simulink model "CtrlStrct_VNT_Level2"  (R2018a)
settings: Solver=VariableStepAuto  StartTime=0.0  StopTime=10.0  FixedStep=sampletime  RelTol=1e-3  EnableMultiTasking=on
PreLoadFcn:
  | Controller_Struct_GoFrom_Scope_1_BusInfo
undefined symbols (not defined in the file or in its folder): canChannel
libraries: canlib x4, canmsglib x4, simulink x1
(part 1 of 2)
settings Model: Creator=IAEC nishito  LastModifiedBy=nishito
settings DataIOCC: LimitDataPoints=on  SaveFormat=Array  SaveOutput=off  SaveTime=off
settings OptimizationCC: DefaultParameterBehavior=Inlined  ExpressionDepthLimit=2147483647  LifeSpan=inf
settings DebuggingCC: UnderspecifiedInitializationDetection=Classic  MergeDetectMultiDrivingBlocksExec=none  SolverPrmCheckMsg=warning  InheritedTsInSrcMsg=none  FcnCallInpInsideContextMsg=warning  StateNameClashWarn=warning  SFUnexpectedBacktrackingDiag=warning  SFNoUnconditionalDefaultTransitionDiag=warning  SFExecutionAtInitializationDiag=none
settings HardwareCC: ProdBitPerPointer=32  ProdBitPerSizeT=32  ProdBitPerPtrDiffT=32  ProdLargestAtomicFloat=None  ProdIntDivRoundTo=Undefined  ProdEndianess=Unspecified  ProdWordSize=32  ProdHWDeviceType=32-bit Generic
settings ModelReferenceCC: ModelReferenceNumInstancesAllowed=Single  PropagateSignalLabelsOutOfModel=off
settings CodeAppCC: StateflowObjectComments=on
settings GRTTargetCC: TargetLangStandard=C89/C90 (ANSI)  GeneratePreprocessorConditionals=Disable all  CombineOutputUpdateFcns=off  GRTInterface=on
settings ConfigComp: CovMetricSettings=dw  CovHtmlReporting=on  CovSaveCumulativeToWorkspaceVar=on  CovSaveSingleToWorkspaceVar=on  CovExternalEMLEnable=off

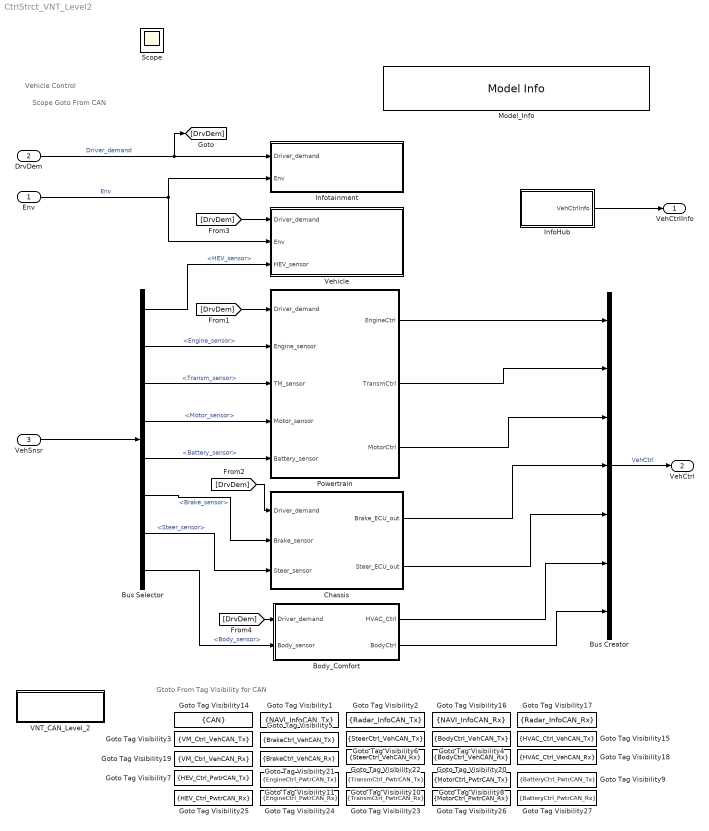
== system CtrlStrct_VNT_Level2 ==
  note: Scope Goto From CAN
  note: Gtoto From Tag Visibility for CAN
  note: Vehicle Control
  Env : Inport  OutDataTypeStr=Bus: Environment_Bus
      settings: AttributesFormatString=<%<OutDataTypeStr>>
  DrvDem : Inport  Port=2  OutDataTypeStr=Bus: Driver_demand_Bus
      settings: AttributesFormatString=%<OutDataTypeStr>
  VehSnsr : Inport  Port=3  OutDataTypeStr=Bus: Vehicle_sensor_Bus
      settings: AttributesFormatString=<%<OutDataTypeStr>>
  Body_Comfort : Subsystem
  Bus Creator : BusCreator  Inputs=7  OutDataTypeStr=Bus: Ctrl_intg_Bus
      settings: AttributesFormatString=%<OutDataTypeStr>
  Bus Selector : BusSelector  OutputSignals=HEV_sensor,Engine_sensor,Transm_sensor,Motor_sensor,Battery_sensor,Brake_sensor,Steer_sensor,Body_sensor
  Chassis : Subsystem
  Goto Tag Visibility1 : GotoTagVisibility  GotoTag=NAVI_InfoCAN_Tx
  Goto Tag Visibility10 : GotoTagVisibility  GotoTag=TransmCtrl_PwtrCAN_Tx
  Goto Tag Visibility11 : GotoTagVisibility  GotoTag=EngineCtrl_PwtrCAN_Tx
  Goto Tag Visibility14 : GotoTagVisibility  GotoTag=CAN
  Goto Tag Visibility15 : GotoTagVisibility  GotoTag=HVAC_Ctrl_VehCAN_Tx
  Goto Tag Visibility16 : GotoTagVisibility  GotoTag=NAVI_InfoCAN_Rx
  Goto Tag Visibility17 : GotoTagVisibility  GotoTag=Radar_InfoCAN_Rx
  Goto Tag Visibility18 : GotoTagVisibility  GotoTag=HVAC_Ctrl_VehCAN_Rx
  Goto Tag Visibility19 : GotoTagVisibility  GotoTag=VM_Ctrl_VehCAN_Rx
  Goto Tag Visibility2 : GotoTagVisibility  GotoTag=Radar_InfoCAN_Tx
  Goto Tag Visibility20 : GotoTagVisibility  GotoTag=BodyCtrl_VehCAN_Rx
  Goto Tag Visibility21 : GotoTagVisibility  GotoTag=BrakeCtrl_VehCAN_Rx
  Goto Tag Visibility22 : GotoTagVisibility  GotoTag=SteerCtrl_VehCAN_Rx
  Goto Tag Visibility23 : GotoTagVisibility  GotoTag=TransmCtrl_PwtrCAN_Rx
  Goto Tag Visibility24 : GotoTagVisibility  GotoTag=EngineCtrl_PwtrCAN_Rx
  Goto Tag Visibility25 : GotoTagVisibility  GotoTag=HEV_Ctrl_PwtrCAN_Rx
  Goto Tag Visibility26 : GotoTagVisibility  GotoTag=MotorCtrl_PwtrCAN_Rx
  Goto Tag Visibility27 : GotoTagVisibility  GotoTag=BatteryCtrl_PwtrCAN_Rx
  Goto Tag Visibility3 : GotoTagVisibility  GotoTag=VM_Ctrl_VehCAN_Tx
  Goto Tag Visibility4 : GotoTagVisibility  GotoTag=BodyCtrl_VehCAN_Tx
  Goto Tag Visibility5 : GotoTagVisibility  GotoTag=BrakeCtrl_VehCAN_Tx
  Goto Tag Visibility6 : GotoTagVisibility  GotoTag=SteerCtrl_VehCAN_Tx
  Goto Tag Visibility7 : GotoTagVisibility  GotoTag=HEV_Ctrl_PwtrCAN_Tx
  Goto Tag Visibility8 : GotoTagVisibility  GotoTag=MotorCtrl_PwtrCAN_Tx
  Goto Tag Visibility9 : GotoTagVisibility  GotoTag=BatteryCtrl_PwtrCAN_Tx
  InfoHub : Subsystem
  Infotainment : Subsystem
  Model_Info : simulink/Model-Wide Utilities/Model Info  Frame=on  DisplayStringWithTags=|  HorizontalTextAlignment=Left  LeftAlignmentValue=0.02
      | Version  %<ModelVersion>
      | LastModifided by %<LastModifiedBy>  Date %<LastModificationDate>
      | Description  %<Description>
  Powertrain : Subsystem
  VNT_CAN_Level_2 : Subsystem  VariantControl=VarObj_CanType_VNT_simu
  Vehicle : Subsystem
  VehCtrlInfo : Outport  OutDataTypeStr=Bus: IntgCtrl_Info_Bus
      settings: AttributesFormatString=<%<OutDataTypeStr>>
  VehCtrl : Outport  Port=2  OutDataTypeStr=Bus: Ctrl_intg_Bus
      settings: AttributesFormatString=<%<OutDataTypeStr>>
  Scope : Scope
  wires:
  InfoHub/1(VehCtrlInfo) -> VehCtrlInfo/1
  Chassis/2(Steer_ECU_out) -> Bus Creator/5
  Env/1 -> Vehicle/2(Env), Infotainment/2(Env)  "Env"
  Bus Creator/1 -> VehCtrl/1  "VehCtrl"
  [DrvDem] -> Powertrain/1(Driver_demand)
  Powertrain/3(MotorCtrl) -> Bus Creator/3
  Bus Selector/3 -> Powertrain/3(TM_sensor)  "<Transm_sensor>"
  Bus Selector/6 -> Chassis/2(Brake_sensor)  "<Brake_sensor>"
  Body_Comfort/2(BodyCtrl) -> Bus Creator/7
  Bus Selector/2 -> Powertrain/2(Engine_sensor)  "<Engine_sensor>"
  Powertrain/2(TransmCtrl) -> Bus Creator/2
  Chassis/1(Brake_ECU_out) -> Bus Creator/4
  VehSnsr/1 -> Bus Selector/1
  [DrvDem] -> Chassis/1(Driver_demand)
  Body_Comfort/1(HVAC_Ctrl) -> Bus Creator/6
  Bus Selector/1 -> Vehicle/3(HEV_sensor)  "<HEV_sensor>"
  Bus Selector/7 -> Chassis/3(Steer_sensor)  "<Steer_sensor>"
  Powertrain/1(EngineCtrl) -> Bus Creator/1
  [DrvDem] -> Vehicle/1(Driver_demand)
  Bus Selector/5 -> Powertrain/5(Battery_sensor)  "<Battery_sensor>"
  DrvDem/1 -> [DrvDem], Infotainment/1(Driver_demand)  "Driver_demand"
  Bus Selector/8 -> Body_Comfort/2(Body_sensor)  "<Body_sensor>"
  Bus Selector/4 -> Powertrain/4(Motor_sensor)  "<Motor_sensor>"
  [DrvDem] -> Body_Comfort/1(Driver_demand)

== system CtrlStrct_VNT_Level2/Body_Comfort ==
  note: Body Control
  Driver_demand : Inport
  Body_sensor : Inport  Port=2
  Body_Control : Subsystem
  HVAC_Control : Subsystem
  HVAC_Ctrl : Outport
  BodyCtrl : Outport  Port=2
  wires:
  Body_Control/1(BodyCtrl) -> BodyCtrl/1
  Driver_demand/1 -> HVAC_Control/1(Driver_demand), Body_Control/1(Driver_demand)
  Body_sensor/1 -> HVAC_Control/2(Body_sensor), Body_Control/2(Body_sensor)
  HVAC_Control/1(HVAC_Ctrl) -> HVAC_Ctrl/1

== system CtrlStrct_VNT_Level2/Chassis ==
  note: Chassis Control
  Driver_demand : Inport
  Brake_sensor : Inport  Port=2
  Steer_sensor : Inport  Port=3
  Brake_Control : Subsystem
  Steer_Control : Subsystem
  Brake_ECU_out : Outport
  Steer_ECU_out : Outport  Port=2
  wires:
  Driver_demand/1 -> Brake_Control/1(Driver_demand), Steer_Control/1(Driver_demand)
  Brake_Control/1(BrakeCtrl) -> Brake_ECU_out/1
  Brake_sensor/1 -> Brake_Control/2(Brake_sensor)
  Steer_Control/1(SteerCtrl) -> Steer_ECU_out/1
  Steer_sensor/1 -> Steer_Control/2(Steer_sensor)

== system CtrlStrct_VNT_Level2/InfoHub ==
  Bus Creator1 : BusCreator  Inputs=2
  Bus Selector : BusSelector  OutputSignals=VehCAN.BrakeCtrl_VehCAN_Tx.BrkCtrl_Vehicle_speed,PwtrCAN.EngineCtrl_PwtrCAN_Tx.EngCtrl_Engine_speed
  Terminator : Terminator
  Terminator1 : Terminator
  VehCtrlInfo : Outport
  wires:
  [HEV_ECU_Info] -> Bus Creator1/1
  [Engine_ECU_Info] -> Bus Creator1/2
  Bus Creator1/1 -> VehCtrlInfo/1  "VehCtrlInfo"
  [CAN] -> Bus Selector/1
  Bus Selector/2 -> Terminator/1  "<EngCtrl_Engine_speed>"
  Bus Selector/1 -> Terminator1/1  "<BrkCtrl_Vehicle_speed>"

== system CtrlStrct_VNT_Level2/Infotainment ==
  note: Infotainment
  Driver_demand : Inport
  Env : Inport  Port=2
  Navigation : Subsystem
  Radar_Detection : Subsystem
  wires:
  Env/1 -> Navigation/2(Env), Radar_Detection/2(Env)
  Driver_demand/1 -> Radar_Detection/1(Driver_demand), Navigation/1(Driver_demand)

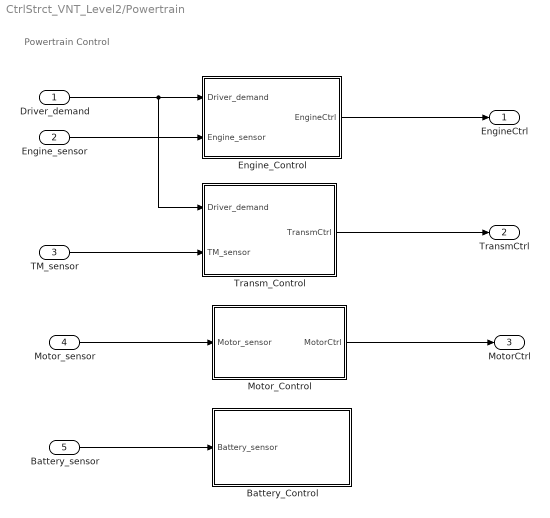
== system CtrlStrct_VNT_Level2/Powertrain ==
  note: Powertrain Control
  Driver_demand : Inport
  Engine_sensor : Inport  Port=2
  TM_sensor : Inport  Port=3
  Motor_sensor : Inport  Port=4
  Battery_sensor : Inport  Port=5
  Battery_Control : Subsystem
  Engine_Control : Subsystem
  Motor_Control : Subsystem
  Transm_Control : Subsystem
  EngineCtrl : Outport
  TransmCtrl : Outport  Port=2
  MotorCtrl : Outport  Port=3
  wires:
  Driver_demand/1 -> Transm_Control/1(Driver_demand), Engine_Control/1(Driver_demand)
  Motor_Control/1(MotorCtrl) -> MotorCtrl/1
  Motor_sensor/1 -> Motor_Control/1(Motor_sensor)
  Battery_sensor/1 -> Battery_Control/1(Battery_sensor)
  Engine_Control/1(EngineCtrl) -> EngineCtrl/1
  Engine_sensor/1 -> Engine_Control/2(Engine_sensor)
  Transm_Control/1(TransmCtrl) -> TransmCtrl/1
  TM_sensor/1 -> Transm_Control/2(TM_sensor)

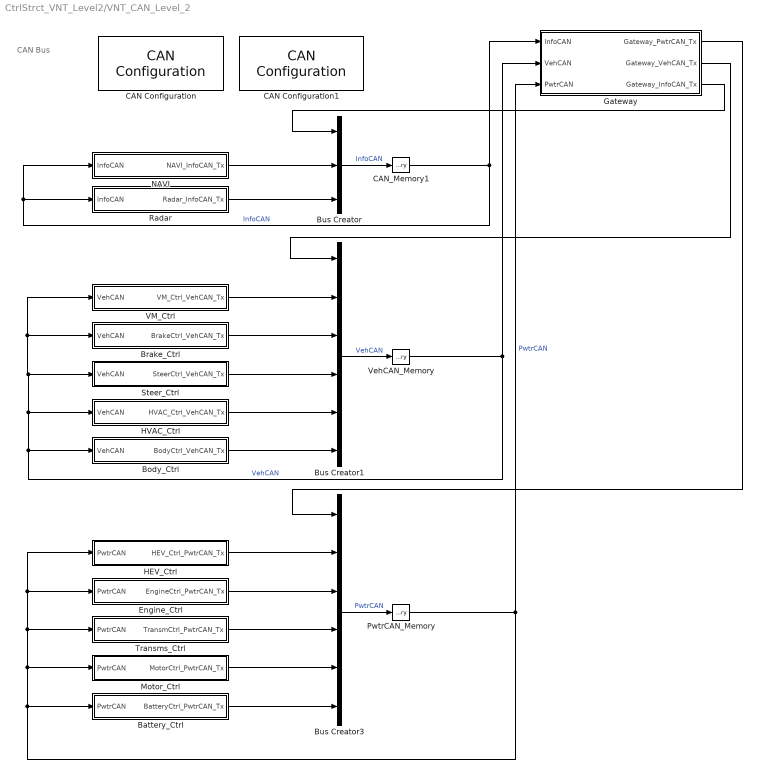
== system CtrlStrct_VNT_Level2/VNT_CAN_Level_2 ==
  note: CAN Bus
  Battery_Ctrl : Subsystem
  Body_Ctrl : Subsystem
  Brake_Ctrl : Subsystem
  Bus Creator : BusCreator  Inputs=3
  Bus Creator1 : BusCreator  Inputs=6
  Bus Creator3 : BusCreator  Inputs=6
  CAN Configuration : canlib/CAN Configuration  BlockHandle=38729.0009  DeviceMenu=MathWorks Virtual 1 (Channel 1)  Device=MathWorks Virtual 1 (Channel 1)  ObjConstructor=canChannel('MathWorks','Virtual 1',1)  BusSpeed=500000  EnableBitParameters=off  AckMode=Normal
      settings: SourceProductName=Vehicle Network Toolbox  SourceProductBaseCode=VN
  CAN Configuration1 : canlib/CAN Configuration  BlockHandle=38730.0009  DeviceMenu=MathWorks Virtual 1 (Channel 2)  Device=MathWorks Virtual 1 (Channel 2)  ObjConstructor=canChannel('MathWorks','Virtual 1',2)  BusSpeed=500000  EnableBitParameters=off  AckMode=Normal
      settings: SourceProductName=Vehicle Network Toolbox  SourceProductBaseCode=VN
  CAN_Memory1 : Memory
  Engine_Ctrl : Subsystem
  Gateway : Subsystem
  HEV_Ctrl : Subsystem
  HVAC_Ctrl : Subsystem
  Motor_Ctrl : Subsystem
  NAVI : Subsystem
  PwtrCAN_Memory : Memory
  Radar : Subsystem
  Steer_Ctrl : Subsystem
  Transms_Ctrl : Subsystem
  VM_Ctrl : Subsystem
  VehCAN_Memory : Memory
  wires:
  Radar/1(Radar_InfoCAN_Tx) -> Bus Creator/3
  NAVI/1(NAVI_InfoCAN_Tx) -> Bus Creator/2
  VM_Ctrl/1(VM_Ctrl_VehCAN_Tx) -> Bus Creator1/2
  Brake_Ctrl/1(BrakeCtrl_VehCAN_Tx) -> Bus Creator1/3
  Steer_Ctrl/1(SteerCtrl_VehCAN_Tx) -> Bus Creator1/4
  HVAC_Ctrl/1(HVAC_Ctrl_VehCAN_Tx) -> Bus Creator1/5
  Body_Ctrl/1(BodyCtrl_VehCAN_Tx) -> Bus Creator1/6
  Battery_Ctrl/1(BatteryCtrl_PwtrCAN_Tx) -> Bus Creator3/6
  Transms_Ctrl/1(TransmCtrl_PwtrCAN_Tx) -> Bus Creator3/4
  Motor_Ctrl/1(MotorCtrl_PwtrCAN_Tx) -> Bus Creator3/5
  Gateway/3(Gateway_InfoCAN_Tx) -> Bus Creator/1
  CAN_Memory1/1 -> NAVI/1(InfoCAN), Radar/1(InfoCAN), Gateway/1(InfoCAN)  "InfoCAN"
  Gateway/2(Gateway_VehCAN_Tx) -> Bus Creator1/1
  Gateway/1(Gateway_PwtrCAN_Tx) -> Bus Creator3/1
  PwtrCAN_Memory/1 -> Motor_Ctrl/1(PwtrCAN), Transms_Ctrl/1(PwtrCAN), Engine_Ctrl/1(PwtrCAN), HEV_Ctrl/1(PwtrCAN), Battery_Ctrl/1(PwtrCAN), Gateway/3(PwtrCAN)  "PwtrCAN"
  VehCAN_Memory/1 -> Body_Ctrl/1(VehCAN), HVAC_Ctrl/1(VehCAN), Brake_Ctrl/1(VehCAN), VM_Ctrl/1(VehCAN), Steer_Ctrl/1(VehCAN), Gateway/2(VehCAN)  "VehCAN"
  HEV_Ctrl/1(HEV_Ctrl_PwtrCAN_Tx) -> Bus Creator3/2
  Engine_Ctrl/1(EngineCtrl_PwtrCAN_Tx) -> Bus Creator3/3
  Bus Creator3/1 -> PwtrCAN_Memory/1  "PwtrCAN"
  Bus Creator/1 -> CAN_Memory1/1  "InfoCAN"
  Bus Creator1/1 -> VehCAN_Memory/1  "VehCAN"

== system CtrlStrct_VNT_Level2/Vehicle ==
  note: Vehicle Integrated Control
  Driver_demand : Inport
  Env : Inport  Port=2
  HEV_sensor : Inport  Port=3
  HEV_Control : Subsystem
  Vehicle_Motion_Control : Subsystem
  wires:
  Env/1 -> Vehicle_Motion_Control/1(Env)
  Driver_demand/1 -> HEV_Control/1(Driver_demand)
  HEV_sensor/1 -> HEV_Control/2(HEV_sensor)

== system CtrlStrct_VNT_Level2/Body_Comfort/Body_Control ==
  note: Body Control
  Driver_demand : Inport
  Body_sensor : Inport  Port=2
  BodyControlModule : ModelReference  ModelNameDialog=BodyCtrl_V1_1.slx  SimulationMode=Normal  ModelReferenceVersion=0.1.16
  Rate Transition1 : RateTransition  Deterministic=off
      settings: AttributesFormatString=<Deterministic=%<Deterministic>>
  Rate Transition2 : RateTransition  Deterministic=off
      settings: AttributesFormatString=<Deterministic=%<Deterministic>>
  Rate Transition4 : RateTransition  Deterministic=off
      settings: AttributesFormatString=<Deterministic=%<Deterministic>>
  BodyCtrl : Outport
  tag scope: BodyCtrl_VehCAN_Tx=scoped
  wires:
  Driver_demand/1 -> Rate Transition2/1
  Rate Transition2/1 -> BodyControlModule/1
  BodyControlModule/1 -> Rate Transition4/1
  [BodyCtrl_VehCAN_Rx] -> BodyControlModule/3
  BodyControlModule/2 -> [BodyCtrl_VehCAN_Tx]  "BodyCtrl_VehCAN_Tx"
  Rate Transition4/1 -> BodyCtrl/1  "BodyCtrl"
  Body_sensor/1 -> Rate Transition1/1
  Rate Transition1/1 -> BodyControlModule/2

== system CtrlStrct_VNT_Level2/Body_Comfort/HVAC_Control ==
  note: HVAC Control
  Driver_demand : Inport
  Body_sensor : Inport  Port=2
  Aircon_Control : ModelReference  ModelNameDialog=HVAC_Ctrl_V1_1.slx  SimulationMode=Normal  ModelReferenceVersion=0.1.22
  Rate Transition1 : RateTransition  Deterministic=off
      settings: AttributesFormatString=<Deterministic=%<Deterministic>>
  Rate Transition2 : RateTransition  Deterministic=off
      settings: AttributesFormatString=<Deterministic=%<Deterministic>>
  Rate Transition4 : RateTransition  Deterministic=off
      settings: AttributesFormatString=<Deterministic=%<Deterministic>>
  HVAC_Ctrl : Outport
  tag scope: HVAC_Ctrl_VehCAN_Tx=scoped
  wires:
  Rate Transition1/1 -> Aircon_Control/2
  Body_sensor/1 -> Rate Transition1/1
  Rate Transition4/1 -> HVAC_Ctrl/1  "HVAC_Ctrl"
  Aircon_Control/2 -> [HVAC_Ctrl_VehCAN_Tx]  "HVAC_Ctrl_VehCAN_Tx"
  [HVAC_Ctrl_VehCAN_Rx] -> Aircon_Control/3
  Aircon_Control/1 -> Rate Transition4/1
  Rate Transition2/1 -> Aircon_Control/1
  Driver_demand/1 -> Rate Transition2/1

== system CtrlStrct_VNT_Level2/Chassis/Brake_Control ==
  note: Brake Control
  Driver_demand : Inport
  Brake_sensor : Inport  Port=2
  Brake_Control : ModelReference  ModelNameDialog=BrakeCtrl_V1_1.slx  SimulationMode=Normal  ModelReferenceVersion=1.0.23
  Rate Transition1 : RateTransition  Deterministic=off
      settings: AttributesFormatString=<Deterministic=%<Deterministic>>
  Rate Transition2 : RateTransition  Deterministic=off
      settings: AttributesFormatString=<Deterministic=%<Deterministic>>
  Rate Transition4 : RateTransition  Deterministic=off
      settings: AttributesFormatString=<Deterministic=%<Deterministic>>
  Terminator : Terminator
  BrakeCtrl : Outport
  tag scope: BrakeCtrl_VehCAN_Tx=scoped
  wires:
  Rate Transition2/1 -> Brake_Control/2
  Driver_demand/1 -> Rate Transition1/1
  Rate Transition1/1 -> Brake_Control/1
  Brake_sensor/1 -> Rate Transition2/1
  Brake_Control/3 -> Terminator/1
  [BrakeCtrl_VehCAN_Rx] -> Brake_Control/3
  Rate Transition4/1 -> BrakeCtrl/1  "BrakeCtrl"
  Brake_Control/1 -> Rate Transition4/1
  Brake_Control/2 -> [BrakeCtrl_VehCAN_Tx]  "BrakeCtrl_VehCAN_Tx"

== system CtrlStrct_VNT_Level2/Chassis/Steer_Control ==
  note: Steering Control
  Driver_demand : Inport
  Steer_sensor : Inport  Port=2
  Rate Transition3 : RateTransition  Deterministic=off
      settings: AttributesFormatString=<Deterministic=%<Deterministic>>
  Rate Transition4 : RateTransition  Deterministic=off
      settings: AttributesFormatString=<Deterministic=%<Deterministic>>
  Rate Transition5 : RateTransition  Deterministic=off
      settings: AttributesFormatString=<Deterministic=%<Deterministic>>
  Steer_Control : ModelReference  ModelNameDialog=SteerCtrl_V1_1.slx  SimulationMode=Normal  ModelReferenceVersion=0.1.16
  SteerCtrl : Outport
  tag scope: SteerCtrl_VehCAN_Tx=scoped
  wires:
  Rate Transition4/1 -> Steer_Control/2
  Driver_demand/1 -> Rate Transition3/1
  Steer_Control/1 -> Rate Transition5/1
  Steer_sensor/1 -> Rate Transition4/1
  [SteerCtrl_VehCAN_Rx] -> Steer_Control/3
  Rate Transition3/1 -> Steer_Control/1
  Rate Transition5/1 -> SteerCtrl/1  "SteerCtrl"
  Steer_Control/2 -> [SteerCtrl_VehCAN_Tx]  "SteerCtrl_VehCAN_Tx"

== system CtrlStrct_VNT_Level2/Infotainment/Navigation ==
  note: Navigation
  Driver_demand : Inport
  Env : Inport  Port=2
  NAVI : ModelReference  ModelNameDialog=NAVI_V1_1.slx  SimulationMode=Normal  ModelReferenceVersion=0.1.17
  Rate Transition1 : RateTransition  Deterministic=off
      settings: AttributesFormatString=<Deterministic=%<Deterministic>>
  Rate Transition4 : RateTransition  Deterministic=off
      settings: AttributesFormatString=<Deterministic=%<Deterministic>>
  tag scope: NAVI_InfoCAN_Tx=scoped
  wires:
  Rate Transition1/1 -> NAVI/1
  Driver_demand/1 -> Rate Transition1/1
  [NAVI_InfoCAN_Rx] -> NAVI/3
  NAVI/1 -> [NAVI_InfoCAN_Tx]  "NAVI_InfoCAN_Tx"
  Env/1 -> Rate Transition4/1
  Rate Transition4/1 -> NAVI/2

== system CtrlStrct_VNT_Level2/Infotainment/Radar_Detection ==
  note: Radar Detection
  Driver_demand : Inport
  Env : Inport  Port=2
  Radar_Detection : ModelReference  ModelNameDialog=Radar_V1_1.slx  SimulationMode=Normal  ModelReferenceVersion=0.1.17
  Rate Transition1 : RateTransition  Deterministic=off
      settings: AttributesFormatString=<Deterministic=%<Deterministic>>
  Rate Transition4 : RateTransition  Deterministic=off
      settings: AttributesFormatString=<Deterministic=%<Deterministic>>
  tag scope: Radar_InfoCAN_Tx=scoped
  wires:
  Rate Transition1/1 -> Radar_Detection/2
  Env/1 -> Rate Transition1/1
  [Radar_InfoCAN_Rx] -> Radar_Detection/3
  Radar_Detection/1 -> [Radar_InfoCAN_Tx]  "Radar_InfoCAN_Tx"
  Driver_demand/1 -> Rate Transition4/1
  Rate Transition4/1 -> Radar_Detection/1

== system CtrlStrct_VNT_Level2/Powertrain/Battery_Control ==
  note: Battery Control
  Battery_sensor : Inport
  Battery_Control : ModelReference  ModelNameDialog=BatteryCtrl_V1_1.slx  SimulationMode=Normal  ModelReferenceVersion=0.1.22
  Rate Transition1 : RateTransition  Deterministic=off
      settings: AttributesFormatString=<Deterministic=%<Deterministic>>
  tag scope: BatteryCtrl_PwtrCAN_Tx=scoped
  wires:
  Battery_sensor/1 -> Rate Transition1/1
  [BatteryCtrl_PwtrCAN_Rx] -> Battery_Control/2
  Rate Transition1/1 -> Battery_Control/1
  Battery_Control/1 -> [BatteryCtrl_PwtrCAN_Tx]  "BatteryCtrl_PwtrCAN_Tx"

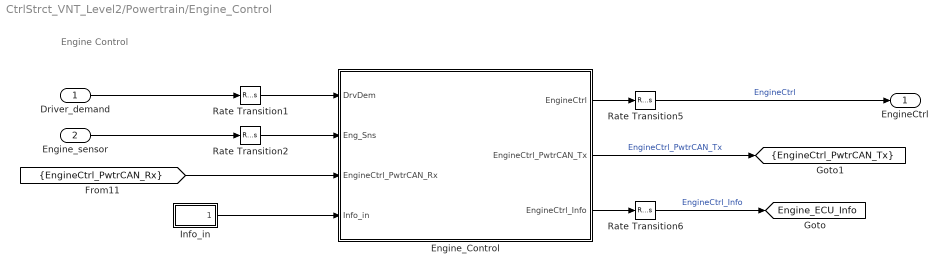
== system CtrlStrct_VNT_Level2/Powertrain/Engine_Control ==
  note: Engine Control
  Driver_demand : Inport
  Engine_sensor : Inport  Port=2
  Engine_Control : Subsystem  Variant=on
  Info_in : Subsystem
  Rate Transition{1..2,5..6} (4 alike) : RateTransition  Deterministic=off
      settings: AttributesFormatString=<Deterministic=%<Deterministic>>
  EngineCtrl : Outport
  tag scope: EngineCtrl_PwtrCAN_Tx=scoped, Engine_ECU_Info=global
  wires:
  Driver_demand/1 -> Rate Transition1/1
  Engine_sensor/1 -> Rate Transition2/1
  Rate Transition5/1 -> EngineCtrl/1  "EngineCtrl"
  Rate Transition6/1 -> [Engine_ECU_Info]  "EngineCtrl_Info"
  Engine_Control/2(" EngineCtrl_PwtrCAN_Tx") -> [EngineCtrl_PwtrCAN_Tx]  "EngineCtrl_PwtrCAN_Tx"
  Rate Transition1/1 -> Engine_Control/1("DrvDem ")
  Rate Transition2/1 -> Engine_Control/2("Eng_Sns ")
  [EngineCtrl_PwtrCAN_Rx] -> Engine_Control/3(EngineCtrl_PwtrCAN_Rx)
  Info_in/1(Info_in) -> Engine_Control/4("Info_in ")
  Engine_Control/1(" EngineCtrl") -> Rate Transition5/1
  Engine_Control/3(" EngineCtrl_Info") -> Rate Transition6/1

== system CtrlStrct_VNT_Level2/Powertrain/Motor_Control ==
  note: Motor Control
  Motor_sensor : Inport
  Motor_Control : ModelReference  ModelNameDialog=MotorCtrl_V1_1.slx  SimulationMode=Normal  ModelReferenceVersion=1.0.21
  Rate Transition1 : RateTransition  Deterministic=off
      settings: AttributesFormatString=<Deterministic=%<Deterministic>>
  Rate Transition3 : RateTransition  Deterministic=off
      settings: AttributesFormatString=<Deterministic=%<Deterministic>>
  Terminator : Terminator
  MotorCtrl : Outport
  tag scope: MotorCtrl_PwtrCAN_Tx=scoped
  wires:
  Rate Transition1/1 -> Motor_Control/1
  [MotorCtrl_PwtrCAN_Rx] -> Motor_Control/2
  Motor_sensor/1 -> Rate Transition1/1
  Motor_Control/3 -> Terminator/1
  Rate Transition3/1 -> MotorCtrl/1  "MotorCtrl"
  Motor_Control/1 -> Rate Transition3/1
  Motor_Control/2 -> [MotorCtrl_PwtrCAN_Tx]  "MotorCtrl_PwtrCAN_Tx"

== system CtrlStrct_VNT_Level2/Powertrain/Transm_Control ==
  note: Transmission Control
  Driver_demand : Inport
  TM_sensor : Inport  Port=2
  Rate Transition3 : RateTransition  Deterministic=off
      settings: AttributesFormatString=<Deterministic=%<Deterministic>>
  Rate Transition4 : RateTransition  Deterministic=off
      settings: AttributesFormatString=<Deterministic=%<Deterministic>>
  Rate Transition5 : RateTransition  Deterministic=off
      settings: AttributesFormatString=<Deterministic=%<Deterministic>>
  Terminator : Terminator
  Transm_ECU : ModelReference  ModelNameDialog=TransmCtrl_V1_1.slx  SimulationMode=Normal  ModelReferenceVersion=1.0.41
  TransmCtrl : Outport
  tag scope: TransmCtrl_PwtrCAN_Tx=scoped
  wires:
  Rate Transition4/1 -> Transm_ECU/2
  Transm_ECU/3 -> Terminator/1
  Driver_demand/1 -> Rate Transition3/1
  TM_sensor/1 -> Rate Transition4/1
  [TransmCtrl_PwtrCAN_Rx] -> Transm_ECU/3
  Rate Transition3/1 -> Transm_ECU/1
  Rate Transition5/1 -> TransmCtrl/1  "TransmCtrl"
  Transm_ECU/1 -> Rate Transition5/1
  Transm_ECU/2 -> [TransmCtrl_PwtrCAN_Tx]  "TransmCtrl_PwtrCAN_Tx"

== system CtrlStrct_VNT_Level2/VNT_CAN_Level_2/Battery_Ctrl ==
  note: Battery control
  note: CAN receive and transmit
  note: Battery Control
  PwtrCAN : Inport
  Bus Creator5 : BusCreator  Inputs=1
  Bus Selector : BusSelector  OutputSignals=HEV_Ctrl_PwtrCAN_Tx.HEVCtrl_Motor_torque_request
  Bus Selector1 : BusSelector  OutputSignals=BatCtrl_SOC
  Rate Transition1 : RateTransition  Deterministic=off
      settings: AttributesFormatString=<Deterministic=%<Deterministic>>
  Rate Transition2 : RateTransition  Deterministic=off
      settings: AttributesFormatString=<Deterministic=%<Deterministic>>
  Terminator : Terminator
  BatteryCtrl_PwtrCAN_Tx : Outport
  tag scope: BatteryCtrl_PwtrCAN_Rx=scoped
  wires:
  Bus Selector/1 -> Bus Creator5/1  "<HEVCtrl_Motor_torque_request>"
  PwtrCAN/1 -> Bus Selector/1
  Bus Creator5/1 -> Rate Transition1/1
  [BatteryCtrl_PwtrCAN_Tx] -> Rate Transition2/1, Bus Selector1/1
  Rate Transition1/1 -> [BatteryCtrl_PwtrCAN_Rx]  "BatteryCtrl_PwtrCAN_Rx"
  Rate Transition2/1 -> BatteryCtrl_PwtrCAN_Tx/1  "BatteryCtrl_PwtrCAN_Tx"
  Bus Selector1/1 -> Terminator/1  "<BatCtrl_SOC>"

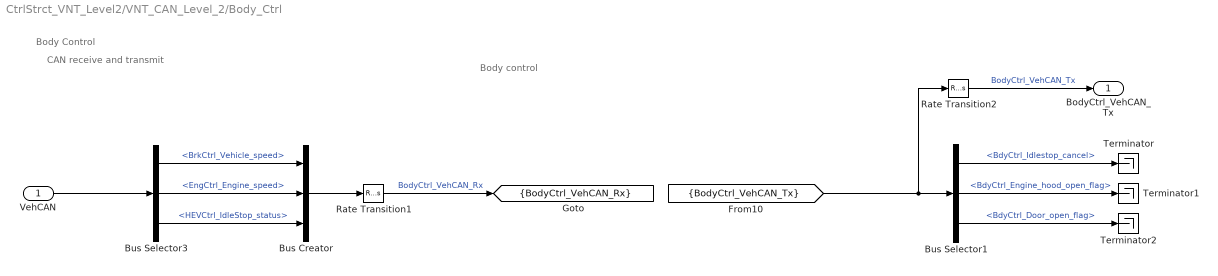
== system CtrlStrct_VNT_Level2/VNT_CAN_Level_2/Body_Ctrl ==
  note: Body Control
  note: CAN receive and transmit
  note: Body control
  VehCAN : Inport
  Bus Creator : BusCreator  Inputs=3
  Bus Selector1 : BusSelector  OutputSignals=BdyCtrl_Idlestop_cancel,BdyCtrl_Engine_hood_open_flag,BdyCtrl_Door_open_flag
  Bus Selector3 : BusSelector  OutputSignals=BrakeCtrl_VehCAN_Tx.BrkCtrl_Vehicle_speed,Gateway_VehCAN_Tx.EngCtrl_Engine_speed,Gateway_VehCAN_Tx.HEVCtrl_IdleStop_status
  Rate Transition1 : RateTransition  Deterministic=off
      settings: AttributesFormatString=<Deterministic=%<Deterministic>>
  Rate Transition2 : RateTransition  Deterministic=off
      settings: AttributesFormatString=<Deterministic=%<Deterministic>>
  Terminator : Terminator
  Terminator1 : Terminator
  Terminator2 : Terminator
  BodyCtrl_VehCAN_Tx : Outport
  tag scope: BodyCtrl_VehCAN_Rx=scoped
  wires:
  Bus Selector1/3 -> Terminator2/1  "<BdyCtrl_Door_open_flag>"
  Bus Selector1/1 -> Terminator/1  "<BdyCtrl_Idlestop_cancel>"
  Bus Selector1/2 -> Terminator1/1  "<BdyCtrl_Engine_hood_open_flag>"
  Rate Transition2/1 -> BodyCtrl_VehCAN_Tx/1  "BodyCtrl_VehCAN_Tx"
  Rate Transition1/1 -> [BodyCtrl_VehCAN_Rx]  "BodyCtrl_VehCAN_Rx"
  [BodyCtrl_VehCAN_Tx] -> Bus Selector1/1, Rate Transition2/1
  VehCAN/1 -> Bus Selector3/1
  Bus Creator/1 -> Rate Transition1/1
  Bus Selector3/2 -> Bus Creator/2  "<EngCtrl_Engine_speed>"
  Bus Selector3/1 -> Bus Creator/1  "<BrkCtrl_Vehicle_speed>"
  Bus Selector3/3 -> Bus Creator/3  "<HEVCtrl_IdleStop_status>"

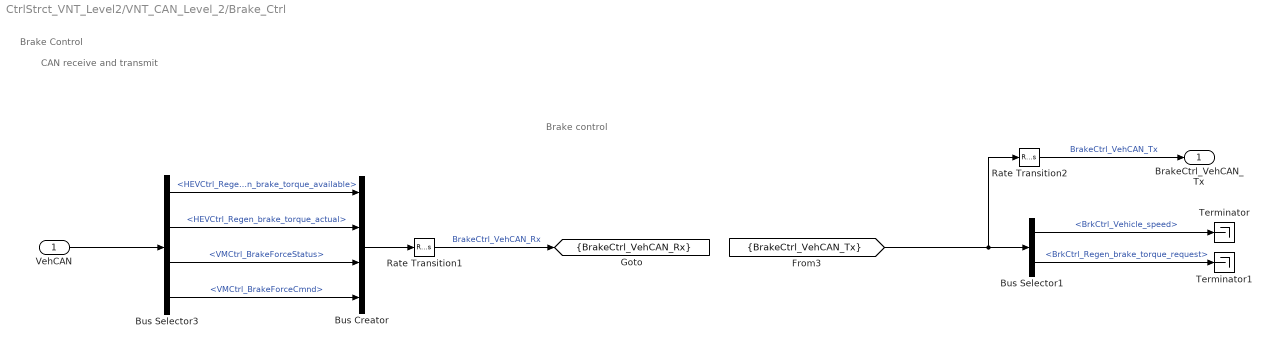
== system CtrlStrct_VNT_Level2/VNT_CAN_Level_2/Brake_Ctrl ==
  note: Brake Control
  note: CAN receive and transmit
  note: Brake control
  VehCAN : Inport
  Bus Creator : BusCreator  Inputs=4
  Bus Selector1 : BusSelector  OutputSignals=BrkCtrl_Vehicle_speed,BrkCtrl_Regen_brake_torque_request
  Bus Selector3 : BusSelector  OutputSignals=Gateway_VehCAN_Tx.HEVCtrl_Regen_brake_torque_available,Gateway_VehCAN_Tx.HEVCtrl_Regen_brake_torque_actual,VM_Ctrl_VehCAN_Tx.VMCtrl_BrakeForceStatus,VM_Ctrl_VehCAN_Tx.VMCtrl_BrakeForceCmnd
  Rate Transition1 : RateTransition  Deterministic=off
      settings: AttributesFormatString=<Deterministic=%<Deterministic>>
  Rate Transition2 : RateTransition  Deterministic=off
      settings: AttributesFormatString=<Deterministic=%<Deterministic>>
  Terminator : Terminator
  Terminator1 : Terminator
  BrakeCtrl_VehCAN_Tx : Outport
  tag scope: BrakeCtrl_VehCAN_Rx=scoped
  wires:
  Bus Selector1/1 -> Terminator/1  "<BrkCtrl_Vehicle_speed>"
  Bus Selector1/2 -> Terminator1/1  "<BrkCtrl_Regen_brake_torque_request>"
  Rate Transition2/1 -> BrakeCtrl_VehCAN_Tx/1  "BrakeCtrl_VehCAN_Tx"
  Rate Transition1/1 -> [BrakeCtrl_VehCAN_Rx]  "BrakeCtrl_VehCAN_Rx"
  [BrakeCtrl_VehCAN_Tx] -> Bus Selector1/1, Rate Transition2/1
  VehCAN/1 -> Bus Selector3/1
  Bus Creator/1 -> Rate Transition1/1
  Bus Selector3/3 -> Bus Creator/3  "<VMCtrl_BrakeForceStatus>"
  Bus Selector3/2 -> Bus Creator/2  "<HEVCtrl_Regen_brake_torque_actual>"
  Bus Selector3/4 -> Bus Creator/4  "<VMCtrl_BrakeForceCmnd>"
  Bus Selector3/1 -> Bus Creator/1  "<HEVCtrl_Regen_brake_torque_available>"

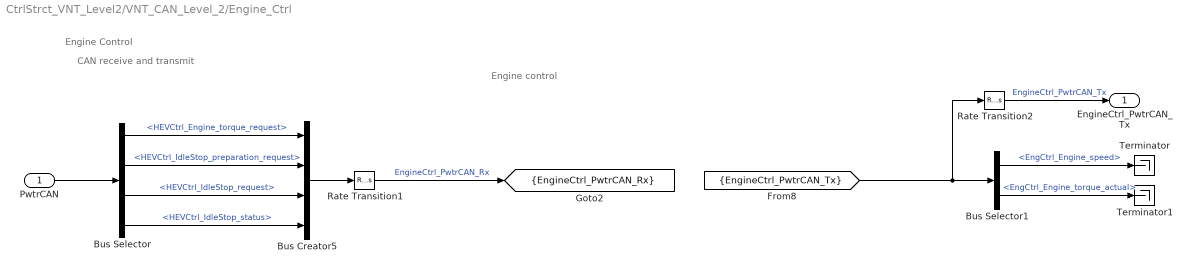
== system CtrlStrct_VNT_Level2/VNT_CAN_Level_2/Engine_Ctrl ==
  note: Engine control
  note: Engine Control
  note: CAN receive and transmit
  PwtrCAN : Inport
  Bus Creator5 : BusCreator  Inputs=4
  Bus Selector : BusSelector  OutputSignals=HEV_Ctrl_PwtrCAN_Tx.HEVCtrl_Engine_torque_request,HEV_Ctrl_PwtrCAN_Tx.HEVCtrl_IdleStop_preparation_request,HEV_Ctrl_PwtrCAN_Tx.HEVCtrl_IdleStop_request,HEV_Ctrl_PwtrCAN_Tx.HEVCtrl_IdleStop_status
  Bus Selector1 : BusSelector  OutputSignals=EngCtrl_Engine_speed,EngCtrl_Engine_torque_actual
  Rate Transition1 : RateTransition  Deterministic=off
      settings: AttributesFormatString=<Deterministic=%<Deterministic>>
  Rate Transition2 : RateTransition  Deterministic=off
      settings: AttributesFormatString=<Deterministic=%<Deterministic>>
  Terminator : Terminator
  Terminator1 : Terminator
  EngineCtrl_PwtrCAN_Tx : Outport
  tag scope: EngineCtrl_PwtrCAN_Rx=scoped
  wires:
  Bus Selector/1 -> Bus Creator5/1  "<HEVCtrl_Engine_torque_request>"
  Bus Selector/3 -> Bus Creator5/3  "<HEVCtrl_IdleStop_request>"
  Bus Selector/4 -> Bus Creator5/4  "<HEVCtrl_IdleStop_status>"
  Bus Selector/2 -> Bus Creator5/2  "<HEVCtrl_IdleStop_preparation_request>"
  [EngineCtrl_PwtrCAN_Tx] -> Rate Transition2/1, Bus Selector1/1
  PwtrCAN/1 -> Bus Selector/1
  Bus Creator5/1 -> Rate Transition1/1
  Rate Transition1/1 -> [EngineCtrl_PwtrCAN_Rx]  "EngineCtrl_PwtrCAN_Rx"
  Rate Transition2/1 -> EngineCtrl_PwtrCAN_Tx/1  "EngineCtrl_PwtrCAN_Tx"
  Bus Selector1/2 -> Terminator1/1  "<EngCtrl_Engine_torque_actual>"
  Bus Selector1/1 -> Terminator/1  "<EngCtrl_Engine_speed>"

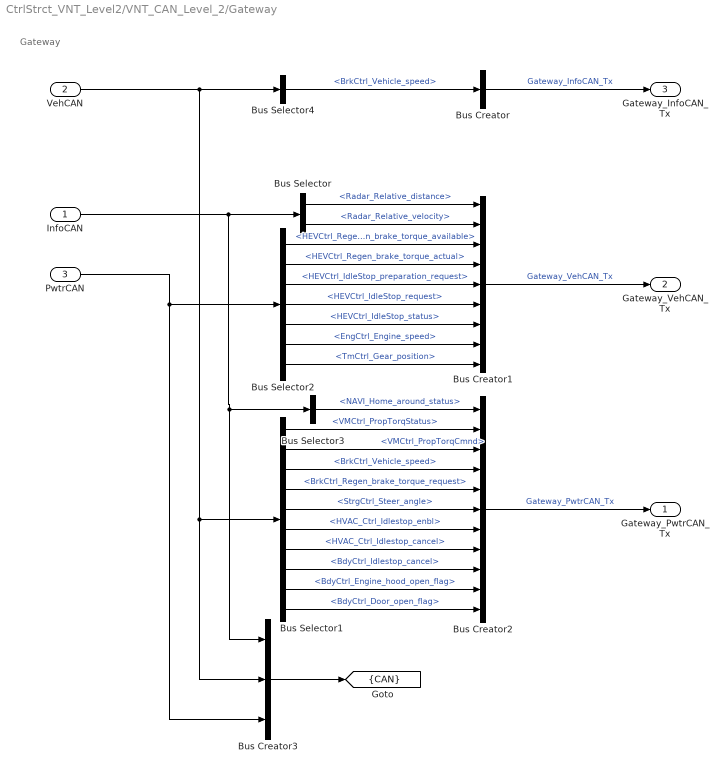
== system CtrlStrct_VNT_Level2/VNT_CAN_Level_2/Gateway ==
  note: Gateway
  InfoCAN : Inport
  VehCAN : Inport  Port=2
  PwtrCAN : Inport  Port=3
  Bus Creator : BusCreator  Inputs=1  OutDataTypeStr=Bus: Gateway_InfoCAN_Tx_Bus
      settings: AttributesFormatString=<%<OutDataTypeStr>>
  Bus Creator1 : BusCreator  Inputs=9  OutDataTypeStr=Bus: Gateway_VehCAN_Tx_Bus
      settings: AttributesFormatString=<%<OutDataTypeStr>>
  Bus Creator2 : BusCreator  Inputs=11  OutDataTypeStr=Bus: Gateway_PwtrCAN_Tx_Bus
      settings: AttributesFormatString=<%<OutDataTypeStr>>
  Bus Creator3 : BusCreator  Inputs=3
  Bus Selector : BusSelector  OutputSignals=Radar_InfoCAN_Tx.Radar_Relative_distance,Radar_InfoCAN_Tx.Radar_Relative_velocity
  Bus Selector1 : BusSelector  OutputSignals=VM_Ctrl_VehCAN_Tx.VMCtrl_PropTorqStatus,VM_Ctrl_VehCAN_Tx.VMCtrl_PropTorqCmnd,BrakeCtrl_VehCAN_Tx.BrkCtrl_Vehicle_speed,BrakeCtrl_VehCAN_Tx.BrkCtrl_Regen_brake_torque_request,SteerCtrl_VehCAN_Tx.StrgCtrl_Steer_angle,HVAC_Ctrl_VehCAN_Tx.HVAC_Ctrl_Idlestop_enbl,HVAC_Ctrl_VehCAN_Tx.HVAC_Ctrl_Idlestop_cancel,BodyCtrl_VehCAN_Tx.BdyCtrl_Idlestop_cancel,BodyCtrl_VehCAN_Tx.BdyCtrl_Engine_hood_open_flag,BodyCtrl_VehCAN_Tx.BdyCtrl_Door_open_flag
  Bus Selector2 : BusSelector  OutputSignals=HEV_Ctrl_PwtrCAN_Tx.HEVCtrl_Regen_brake_torque_available,HEV_Ctrl_PwtrCAN_Tx.HEVCtrl_Regen_brake_torque_actual,HEV_Ctrl_PwtrCAN_Tx.HEVCtrl_IdleStop_preparation_request,HEV_Ctrl_PwtrCAN_Tx.HEVCtrl_IdleStop_request,HEV_Ctrl_PwtrCAN_Tx.HEVCtrl_IdleStop_status,EngineCtrl_PwtrCAN_Tx.EngCtrl_Engine_speed,TransmCtrl_PwtrCAN_Tx.TmCtrl_Gear_position
  Bus Selector3 : BusSelector  OutputSignals=NAVI_InfoCAN_Tx.NAVI_Home_around_status
  Bus Selector4 : BusSelector  OutputSignals=BrakeCtrl_VehCAN_Tx.BrkCtrl_Vehicle_speed
  Gateway_PwtrCAN_Tx : Outport
  Gateway_VehCAN_Tx : Outport  Port=2
  Gateway_InfoCAN_Tx : Outport  Port=3
  tag scope: CAN=scoped
  wires:
  Bus Creator3/1 -> [CAN]
  Bus Creator/1 -> Gateway_InfoCAN_Tx/1  "Gateway_InfoCAN_Tx"
  Bus Selector4/1 -> Bus Creator/1  "<BrkCtrl_Vehicle_speed>"
  Bus Selector2/7 -> Bus Creator1/9  "<TmCtrl_Gear_position>"
  Bus Selector2/6 -> Bus Creator1/8  "<EngCtrl_Engine_speed>"
  Bus Selector2/2 -> Bus Creator1/4  "<HEVCtrl_Regen_brake_torque_actual>"
  Bus Selector2/1 -> Bus Creator1/3  "<HEVCtrl_Regen_brake_torque_available>"
  Bus Creator2/1 -> Gateway_PwtrCAN_Tx/1  "Gateway_PwtrCAN_Tx"
  Bus Selector1/10 -> Bus Creator2/11  "<BdyCtrl_Door_open_flag>"
  Bus Selector1/9 -> Bus Creator2/10  "<BdyCtrl_Engine_hood_open_flag>"
  Bus Selector1/8 -> Bus Creator2/9  "<BdyCtrl_Idlestop_cancel>"
  Bus Selector1/7 -> Bus Creator2/8  "<HVAC_Ctrl_Idlestop_cancel>"
  Bus Selector1/6 -> Bus Creator2/7  "<HVAC_Ctrl_Idlestop_enbl>"
  Bus Selector1/5 -> Bus Creator2/6  "<StrgCtrl_Steer_angle>"
  Bus Selector1/4 -> Bus Creator2/5  "<BrkCtrl_Regen_brake_torque_request>"
  Bus Selector1/3 -> Bus Creator2/4  "<BrkCtrl_Vehicle_speed>"
  Bus Selector3/1 -> Bus Creator2/1  "<NAVI_Home_around_status>"
  Bus Selector/2 -> Bus Creator1/2  "<Radar_Relative_velocity>"
  Bus Selector/1 -> Bus Creator1/1  "<Radar_Relative_distance>"
  InfoCAN/1 -> Bus Selector/1, Bus Selector3/1, Bus Creator3/1
  PwtrCAN/1 -> Bus Creator3/3, Bus Selector2/1
  Bus Creator1/1 -> Gateway_VehCAN_Tx/1  "Gateway_VehCAN_Tx"
  VehCAN/1 -> Bus Selector4/1, Bus Selector1/1, Bus Creator3/2
  Bus Selector1/1 -> Bus Creator2/2  "<VMCtrl_PropTorqStatus>"
  Bus Selector1/2 -> Bus Creator2/3  "<VMCtrl_PropTorqCmnd>"
  Bus Selector2/3 -> Bus Creator1/5  "<HEVCtrl_IdleStop_preparation_request>"
  Bus Selector2/4 -> Bus Creator1/6  "<HEVCtrl_IdleStop_request>"
  Bus Selector2/5 -> Bus Creator1/7  "<HEVCtrl_IdleStop_status>"

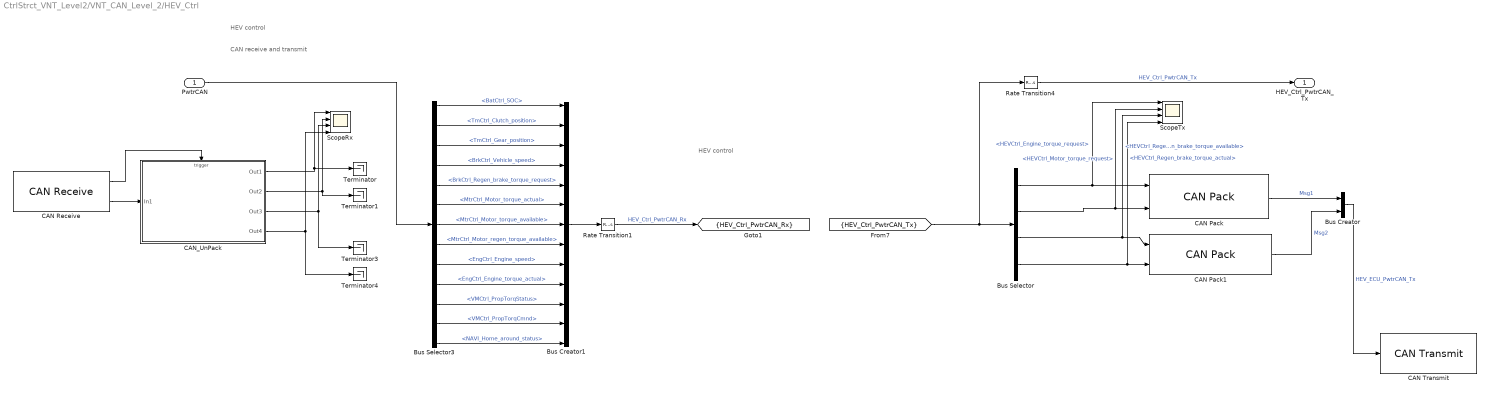
== system CtrlStrct_VNT_Level2/VNT_CAN_Level_2/HEV_Ctrl ==
  note: HEV control
  note: HEV control
  note: CAN receive and transmit
  PwtrCAN : Inport
  Bus Creator : BusCreator  Inputs=2
  Bus Creator1 : BusCreator  Inputs=13
  Bus Selector : BusSelector  OutputSignals=HEVCtrl_Engine_torque_request,HEVCtrl_Motor_torque_request,HEVCtrl_Regen_brake_torque_available,HEVCtrl_Regen_brake_torque_actual
  Bus Selector3 : BusSelector  OutputSignals=BatteryCtrl_PwtrCAN_Tx.BatCtrl_SOC,TransmCtrl_PwtrCAN_Tx.TmCtrl_Clutch_position,TransmCtrl_PwtrCAN_Tx.TmCtrl_Gear_position,Gateway_PwtrCAN_Tx.BrkCtrl_Vehicle_speed,Gateway_PwtrCAN_Tx.BrkCtrl_Regen_brake_torque_request,MotorCtrl_PwtrCAN_Tx.MtrCtrl_Motor_torque_actual,MotorCtrl_PwtrCAN_Tx.MtrCtrl_Motor_torque_available,MotorCtrl_PwtrCAN_Tx.MtrCtrl_Motor_regen_torque_available,EngineCtrl_PwtrCAN_Tx.EngCtrl_Engine_speed,EngineCtrl_PwtrCAN_Tx.EngCtrl_Engine_torque_actual,Gateway_PwtrCAN_Tx.VMCtrl_PropTorqStatus,Gateway_PwtrCAN_Tx.VMCtrl_PropTorqCmnd,Gateway_PwtrCAN_Tx.NAVI_Home_around_status
  CAN Pack : canmsglib/CAN Pack  MsgList=(none)  MsgName=CAN Msg1  MsgIDType=Standard (11-bit identifier)  MsgIdentifier=10  MsgLength=8  SignalInfo=Signal1$0$32$1$3$1$0$1$0$-Inf$Inf$#Signal2$32$32$1$3$1$0$1$0$-Inf$Inf$#  NSignals=2  StartBits=str2num('[int32(0);int32(32)]')  SignalSizes=str2num('[int32(32);int32(32)]')  ByteOrders=str2num('[int32(1);int32(1)]')  DataTypes=str2num('[int32(3);int32(3)]')  MultiplexTypes=str2num('[int32(1);int32(1)]')  MultiplexValues=str2num('[double(0);double(0)]')  Factors=str2num('[double(1);double(1)]')  Offsets=str2num('[double(0);double(0)]')  Minimums=str2num('[double(-Inf);double(-Inf)]')  Maximums=str2num('[double(Inf);double(Inf)]')  Remote=off  ApplyMinMax=off  BusOutput=off
      settings: SourceProductName=Simulink Real-Time  SourceProductBaseCode=XP  DataFormat=manually specified signals
  CAN Pack1 : canmsglib/CAN Pack  MsgList=(none)  MsgName=CAN Msg2  MsgIDType=Standard (11-bit identifier)  MsgIdentifier=20  MsgLength=8  SignalInfo=Signal1$0$32$1$3$1$0$1$0$-Inf$Inf$#Signal2$32$32$1$3$1$0$1$0$-Inf$Inf$#  NSignals=2  StartBits=str2num('[int32(0);int32(32)]')  SignalSizes=str2num('[int32(32);int32(32)]')  ByteOrders=str2num('[int32(1);int32(1)]')  DataTypes=str2num('[int32(3);int32(3)]')  MultiplexTypes=str2num('[int32(1);int32(1)]')  MultiplexValues=str2num('[double(0);double(0)]')  Factors=str2num('[double(1);double(1)]')  Offsets=str2num('[double(0);double(0)]')  Minimums=str2num('[double(-Inf);double(-Inf)]')  Maximums=str2num('[double(Inf);double(Inf)]')  Remote=off  ApplyMinMax=off  BusOutput=off
      settings: SourceProductName=Simulink Real-Time  SourceProductBaseCode=XP  DataFormat=manually specified signals
  CAN Receive : canlib/CAN Receive  BlockHandle=38824.0009  DeviceMenu=MathWorks Virtual 1 (Channel 1)  Device=MathWorks Virtual 1 (Channel 1)  ObjConstructor=canChannel('MathWorks','Virtual 1',1)  EnableStandardIDsFilter=off  StandardIDs=0  EnableExtendedIDsFilter=off  ExtendedIDs=0  SampleTime=0.01  MsgsPerTimestep=all  StdIDsCombo=Allow all  ExtIDsCombo=Allow all  InternalFilterUpdateStatus=off  BusOutput=off
      settings: SourceProductName=Vehicle Network Toolbox  SourceProductBaseCode=VN
  CAN Transmit : canlib/CAN Transmit  BlockHandle=38825.0009  DeviceMenu=MathWorks Virtual 1 (Channel 1)  Device=MathWorks Virtual 1 (Channel 1)  ObjConstructor=canChannel('MathWorks','Virtual 1',1)  EnablePeriodicTransmit=on  MessagePeriod=0.01
      settings: SourceProductName=Vehicle Network Toolbox  SourceProductBaseCode=VN
  CAN_UnPack : Subsystem
  Rate Transition1 : RateTransition  Deterministic=off
      settings: AttributesFormatString=<Deterministic=%<Deterministic>>
  Rate Transition4 : RateTransition  Deterministic=off
      settings: AttributesFormatString=<Deterministic=%<Deterministic>>
  ScopeRx : Scope  NumInputPorts=4
  ScopeTx : Scope  NumInputPorts=4
  Terminator{,1,3..4} (4 alike) : Terminator
  HEV_Ctrl_PwtrCAN_Tx : Outport
  tag scope: HEV_Ctrl_PwtrCAN_Rx=scoped
  wires:
  Bus Selector3/1 -> Bus Creator1/1  "<BatCtrl_SOC>"
  Bus Selector3/9 -> Bus Creator1/9  "<EngCtrl_Engine_speed>"
  Bus Selector3/8 -> Bus Creator1/8  "<MtrCtrl_Motor_regen_torque_available>"
  Bus Selector3/3 -> Bus Creator1/3  "<TmCtrl_Gear_position>"
  PwtrCAN/1 -> Bus Selector3/1
  Bus Selector3/6 -> Bus Creator1/6  "<MtrCtrl_Motor_torque_actual>"
  Bus Selector3/10 -> Bus Creator1/10  "<EngCtrl_Engine_torque_actual>"
  Bus Selector3/4 -> Bus Creator1/4  "<BrkCtrl_Vehicle_speed>"
  Bus Selector3/2 -> Bus Creator1/2  "<TmCtrl_Clutch_position>"
  Bus Selector3/7 -> Bus Creator1/7  "<MtrCtrl_Motor_torque_available>"
  Bus Selector3/5 -> Bus Creator1/5  "<BrkCtrl_Regen_brake_torque_request>"
  Bus Selector3/12 -> Bus Creator1/12  "<VMCtrl_PropTorqCmnd>"
  Bus Selector3/13 -> Bus Creator1/13  "<NAVI_Home_around_status>"
  Bus Selector3/11 -> Bus Creator1/11  "<VMCtrl_PropTorqStatus>"
  CAN Receive/1 -> CAN_UnPack/Trigger
  CAN Receive/2 -> CAN_UnPack/1(In1)
  CAN_UnPack/1(Out1) -> ScopeRx/1, Terminator/1
  CAN_UnPack/2(Out2) -> ScopeRx/2, Terminator1/1
  CAN_UnPack/4(Out4) -> ScopeRx/4, Terminator4/1
  CAN_UnPack/3(Out3) -> ScopeRx/3, Terminator3/1
  Bus Creator1/1 -> Rate Transition1/1
  Bus Creator/1 -> CAN Transmit/1  "HEV_ECU_PwtrCAN_Tx"
  CAN Pack1/1 -> Bus Creator/2  "Msg2"
  CAN Pack/1 -> Bus Creator/1  "Msg1"
  Bus Selector/4 -> CAN Pack1/2, ScopeTx/4  "<HEVCtrl_Regen_brake_torque_actual>"
  Bus Selector/3 -> ScopeTx/3, CAN Pack1/1  "<HEVCtrl_Regen_brake_torque_available>"
  Bus Selector/2 -> ScopeTx/2, CAN Pack/2  "<HEVCtrl_Motor_torque_request>"
  Bus Selector/1 -> ScopeTx/1, CAN Pack/1  "<HEVCtrl_Engine_torque_request>"
  [HEV_Ctrl_PwtrCAN_Tx] -> Rate Transition4/1, Bus Selector/1
  Rate Transition4/1 -> HEV_Ctrl_PwtrCAN_Tx/1  "HEV_Ctrl_PwtrCAN_Tx"
  Rate Transition1/1 -> [HEV_Ctrl_PwtrCAN_Rx]  "HEV_Ctrl_PwtrCAN_Rx"

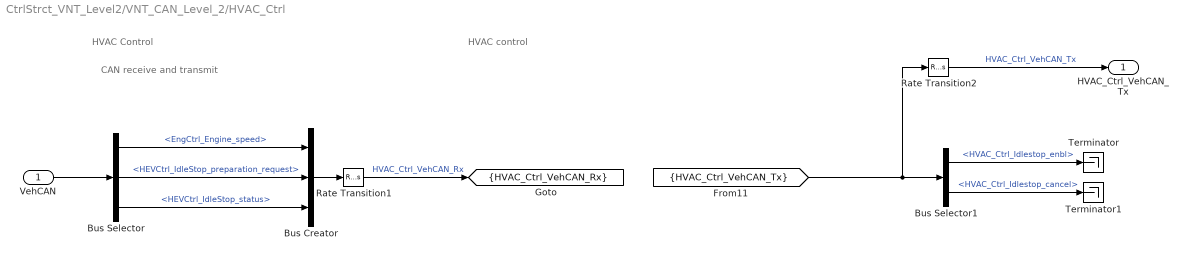
== system CtrlStrct_VNT_Level2/VNT_CAN_Level_2/HVAC_Ctrl ==
  note: HVAC Control
  note: CAN receive and transmit
  note: HVAC control
  VehCAN : Inport
  Bus Creator : BusCreator  Inputs=3
  Bus Selector : BusSelector  OutputSignals=Gateway_VehCAN_Tx.EngCtrl_Engine_speed,Gateway_VehCAN_Tx.HEVCtrl_IdleStop_preparation_request,Gateway_VehCAN_Tx.HEVCtrl_IdleStop_status
  Bus Selector1 : BusSelector  OutputSignals=HVAC_Ctrl_Idlestop_enbl,HVAC_Ctrl_Idlestop_cancel
  Rate Transition1 : RateTransition  Deterministic=off
      settings: AttributesFormatString=<Deterministic=%<Deterministic>>
  Rate Transition2 : RateTransition  Deterministic=off
      settings: AttributesFormatString=<Deterministic=%<Deterministic>>
  Terminator : Terminator
  Terminator1 : Terminator
  HVAC_Ctrl_VehCAN_Tx : Outport
  tag scope: HVAC_Ctrl_VehCAN_Rx=scoped
  wires:
  Bus Selector1/2 -> Terminator1/1  "<HVAC_Ctrl_Idlestop_cancel>"
  Bus Selector1/1 -> Terminator/1  "<HVAC_Ctrl_Idlestop_enbl>"
  Rate Transition2/1 -> HVAC_Ctrl_VehCAN_Tx/1  "HVAC_Ctrl_VehCAN_Tx"
  Rate Transition1/1 -> [HVAC_Ctrl_VehCAN_Rx]  "HVAC_Ctrl_VehCAN_Rx"
  [HVAC_Ctrl_VehCAN_Tx] -> Bus Selector1/1, Rate Transition2/1
  VehCAN/1 -> Bus Selector/1
  Bus Creator/1 -> Rate Transition1/1
  Bus Selector/3 -> Bus Creator/3  "<HEVCtrl_IdleStop_status>"
  Bus Selector/2 -> Bus Creator/2  "<HEVCtrl_IdleStop_preparation_request>"
  Bus Selector/1 -> Bus Creator/1  "<EngCtrl_Engine_speed>"

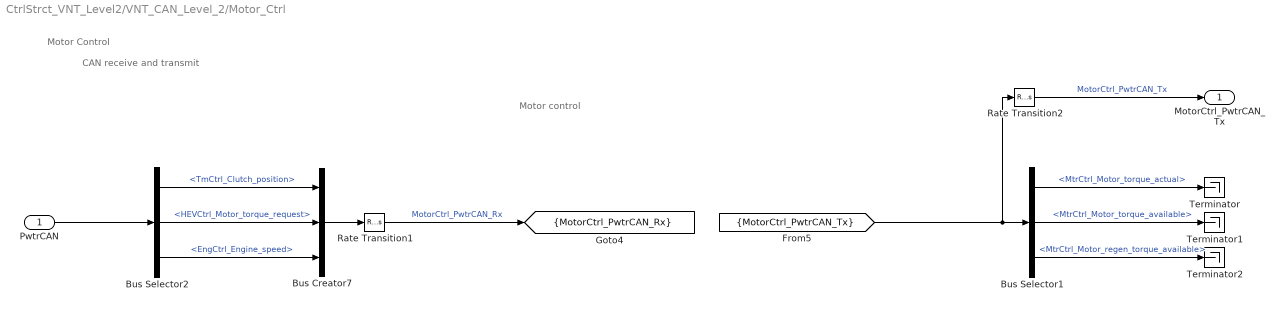
== system CtrlStrct_VNT_Level2/VNT_CAN_Level_2/Motor_Ctrl ==
  note: Motor control
  note: Motor Control
  note: CAN receive and transmit
  PwtrCAN : Inport
  Bus Creator7 : BusCreator  Inputs=3
  Bus Selector1 : BusSelector  OutputSignals=MtrCtrl_Motor_torque_actual,MtrCtrl_Motor_torque_available,MtrCtrl_Motor_regen_torque_available
  Bus Selector2 : BusSelector  OutputSignals=TransmCtrl_PwtrCAN_Tx.TmCtrl_Clutch_position,HEV_Ctrl_PwtrCAN_Tx.HEVCtrl_Motor_torque_request,EngineCtrl_PwtrCAN_Tx.EngCtrl_Engine_speed
  Rate Transition1 : RateTransition  Deterministic=off
      settings: AttributesFormatString=<Deterministic=%<Deterministic>>
  Rate Transition2 : RateTransition  Deterministic=off
      settings: AttributesFormatString=<Deterministic=%<Deterministic>>
  Terminator : Terminator
  Terminator1 : Terminator
  Terminator2 : Terminator
  MotorCtrl_PwtrCAN_Tx : Outport
  tag scope: MotorCtrl_PwtrCAN_Rx=scoped
  wires:
  [MotorCtrl_PwtrCAN_Tx] -> Bus Selector1/1, Rate Transition2/1
  Rate Transition1/1 -> [MotorCtrl_PwtrCAN_Rx]  "MotorCtrl_PwtrCAN_Rx"
  Bus Selector2/2 -> Bus Creator7/2  "<HEVCtrl_Motor_torque_request>"
  Bus Creator7/1 -> Rate Transition1/1
  Bus Selector2/3 -> Bus Creator7/3  "<EngCtrl_Engine_speed>"
  Bus Selector2/1 -> Bus Creator7/1  "<TmCtrl_Clutch_position>"
  Rate Transition2/1 -> MotorCtrl_PwtrCAN_Tx/1  "MotorCtrl_PwtrCAN_Tx"
  PwtrCAN/1 -> Bus Selector2/1
  Bus Selector1/1 -> Terminator/1  "<MtrCtrl_Motor_torque_actual>"
  Bus Selector1/2 -> Terminator1/1  "<MtrCtrl_Motor_torque_available>"
  Bus Selector1/3 -> Terminator2/1  "<MtrCtrl_Motor_regen_torque_available>"

== system CtrlStrct_VNT_Level2/VNT_CAN_Level_2/NAVI ==
  note: Navigation
  note: CAN receive and transmit
  note: Navigation
  InfoCAN : Inport
  Bus Creator : BusCreator  Inputs=1
  Bus Selector1 : BusSelector  OutputSignals=Gateway_InfoCAN_Tx.BrkCtrl_Vehicle_speed
  Bus Selector2 : BusSelector  OutputSignals=NAVI_Road_information,NAVI_Home_around_status
  Rate Transition1 : RateTransition  Deterministic=off
      settings: AttributesFormatString=<Deterministic=%<Deterministic>>
  Rate Transition2 : RateTransition  Deterministic=off
      settings: AttributesFormatString=<Deterministic=%<Deterministic>>
  Terminator : Terminator
  Terminator1 : Terminator
  NAVI_InfoCAN_Tx : Outport
  tag scope: NAVI_InfoCAN_Rx=scoped
  wires:
  Bus Creator/1 -> Rate Transition1/1
  Bus Selector1/1 -> Bus Creator/1  "<BrkCtrl_Vehicle_speed>"
  InfoCAN/1 -> Bus Selector1/1
  [NAVI_InfoCAN_Tx] -> Rate Transition2/1, Bus Selector2/1
  Rate Transition1/1 -> [NAVI_InfoCAN_Rx]  "NAVI_InfoCAN_Rx"
  Rate Transition2/1 -> NAVI_InfoCAN_Tx/1  "NAVI_InfoCAN_Tx"
  Bus Selector2/1 -> Terminator/1  "<NAVI_Road_information>"
  Bus Selector2/2 -> Terminator1/1  "<NAVI_Home_around_status>"

== system CtrlStrct_VNT_Level2/VNT_CAN_Level_2/Radar ==
  note: Radar detection
  note: CAN receive and transmit
  note: Radar Detection
  InfoCAN : Inport
  Bus Creator : BusCreator  Inputs=1
  Bus Selector1 : BusSelector  OutputSignals=Gateway_InfoCAN_Tx.BrkCtrl_Vehicle_speed
  Bus Selector2 : BusSelector  OutputSignals=Radar_Relative_distance,Radar_Relative_velocity
  Rate Transition1 : RateTransition  Deterministic=off
      settings: AttributesFormatString=<Deterministic=%<Deterministic>>
  Rate Transition2 : RateTransition  Deterministic=off
      settings: AttributesFormatString=<Deterministic=%<Deterministic>>
  Terminator : Terminator
  Terminator1 : Terminator
  Radar_InfoCAN_Tx : Outport
  tag scope: Radar_InfoCAN_Rx=scoped
  wires:
  InfoCAN/1 -> Bus Selector1/1
  Bus Creator/1 -> Rate Transition1/1
  Bus Selector1/1 -> Bus Creator/1  "<BrkCtrl_Vehicle_speed>"
  [Radar_InfoCAN_Tx] -> Rate Transition2/1, Bus Selector2/1
  Rate Transition1/1 -> [Radar_InfoCAN_Rx]  "Radar_InfoCAN_Rx"
  Rate Transition2/1 -> Radar_InfoCAN_Tx/1  "Radar_InfoCAN_Tx"
  Bus Selector2/1 -> Terminator/1  "<Radar_Relative_distance>"
  Bus Selector2/2 -> Terminator1/1  "<Radar_Relative_velocity>"

== system CtrlStrct_VNT_Level2/VNT_CAN_Level_2/Steer_Ctrl ==
  note: Steering control
  note: CAN receive and transmit
  note: Steering Control
  VehCAN : Inport
  Bus Creator : BusCreator  Inputs=1
  Bus Selector1 : BusSelector  OutputSignals=BrakeCtrl_VehCAN_Tx.BrkCtrl_Vehicle_speed
  Bus Selector2 : BusSelector  OutputSignals=StrgCtrl_Steer_angle
  Rate Transition1 : RateTransition  Deterministic=off
      settings: AttributesFormatString=<Deterministic=%<Deterministic>>
  Rate Transition2 : RateTransition  Deterministic=off
      settings: AttributesFormatString=<Deterministic=%<Deterministic>>
  Terminator : Terminator
  SteerCtrl_VehCAN_Tx : Outport
  tag scope: SteerCtrl_VehCAN_Rx=scoped
  wires:
  Bus Creator/1 -> Rate Transition1/1
  Bus Selector1/1 -> Bus Creator/1  "<BrkCtrl_Vehicle_speed>"
  VehCAN/1 -> Bus Selector1/1
  [SteerCtrl_VehCAN_Tx] -> Bus Selector2/1, Rate Transition2/1
  Rate Transition1/1 -> [SteerCtrl_VehCAN_Rx]  "SteerCtrl_VehCAN_Rx"
  Rate Transition2/1 -> SteerCtrl_VehCAN_Tx/1  "SteerCtrl_VehCAN_Tx"
  Bus Selector2/1 -> Terminator/1  "<StrgCtrl_Steer_angle>"

== system CtrlStrct_VNT_Level2/VNT_CAN_Level_2/Transms_Ctrl ==
  note: Transmission control
  note: CAN receive and transmit
  note: Transmission Control
  PwtrCAN : Inport
  Bus Creator6 : BusCreator  Inputs=2
  Bus Selector1 : BusSelector  OutputSignals=Gateway_PwtrCAN_Tx.BrkCtrl_Vehicle_speed,EngineCtrl_PwtrCAN_Tx.EngCtrl_Engine_speed
  Bus Selector2 : BusSelector  OutputSignals=TmCtrl_Clutch_position,TmCtrl_Gear_position
  Rate Transition1 : RateTransition  Deterministic=off
      settings: AttributesFormatString=<Deterministic=%<Deterministic>>
  Rate Transition2 : RateTransition  Deterministic=off
      settings: AttributesFormatString=<Deterministic=%<Deterministic>>
  Terminator : Terminator
  Terminator1 : Terminator
  TransmCtrl_PwtrCAN_Tx : Outport
  tag scope: TransmCtrl_PwtrCAN_Rx=scoped
  wires:
  [TransmCtrl_PwtrCAN_Tx] -> Rate Transition2/1, Bus Selector2/1
  Rate Transition2/1 -> TransmCtrl_PwtrCAN_Tx/1  "TransmCtrl_PwtrCAN_Tx"
  Bus Creator6/1 -> Rate Transition1/1
  Bus Selector1/2 -> Bus Creator6/2  "<EngCtrl_Engine_speed>"
  Bus Selector1/1 -> Bus Creator6/1  "<BrkCtrl_Vehicle_speed>"
  PwtrCAN/1 -> Bus Selector1/1
  Rate Transition1/1 -> [TransmCtrl_PwtrCAN_Rx]  "TransmCtrl_PwtrCAN_Rx"
  Bus Selector2/1 -> Terminator/1  "<TmCtrl_Clutch_position>"
  Bus Selector2/2 -> Terminator1/1  "<TmCtrl_Gear_position>"

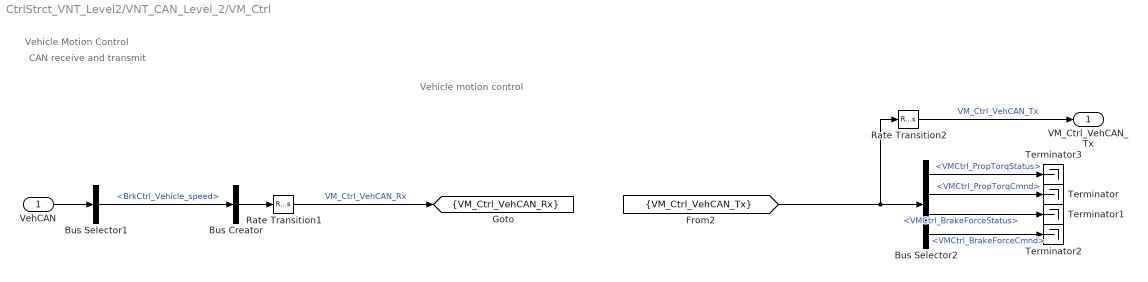
== system CtrlStrct_VNT_Level2/VNT_CAN_Level_2/VM_Ctrl ==
  note: Vehicle motion control
  note: Vehicle Motion Control
  note: CAN receive and transmit
  VehCAN : Inport
  Bus Creator : BusCreator  Inputs=1
  Bus Selector1 : BusSelector  OutputSignals=BrakeCtrl_VehCAN_Tx.BrkCtrl_Vehicle_speed
  Bus Selector2 : BusSelector  OutputSignals=VMCtrl_PropTorqStatus,VMCtrl_PropTorqCmnd,VMCtrl_BrakeForceStatus,VMCtrl_BrakeForceCmnd
  Rate Transition1 : RateTransition  Deterministic=off
      settings: AttributesFormatString=<Deterministic=%<Deterministic>>
  Rate Transition2 : RateTransition  Deterministic=off
      settings: AttributesFormatString=<Deterministic=%<Deterministic>>
  Terminator{,1..3} (4 alike) : Terminator
  VM_Ctrl_VehCAN_Tx : Outport
  tag scope: VM_Ctrl_VehCAN_Rx=scoped
  wires:
  Bus Selector2/4 -> Terminator2/1  "<VMCtrl_BrakeForceCmnd>"
  Bus Selector2/3 -> Terminator1/1  "<VMCtrl_BrakeForceStatus>"
  Bus Selector2/1 -> Terminator3/1  "<VMCtrl_PropTorqStatus>"
  Bus Creator/1 -> Rate Transition1/1
  Bus Selector1/1 -> Bus Creator/1  "<BrkCtrl_Vehicle_speed>"
  VehCAN/1 -> Bus Selector1/1
  [VM_Ctrl_VehCAN_Tx] -> Rate Transition2/1, Bus Selector2/1
  Rate Transition1/1 -> [VM_Ctrl_VehCAN_Rx]  "VM_Ctrl_VehCAN_Rx"
  Rate Transition2/1 -> VM_Ctrl_VehCAN_Tx/1  "VM_Ctrl_VehCAN_Tx"
  Bus Selector2/2 -> Terminator/1  "<VMCtrl_PropTorqCmnd>"

== system CtrlStrct_VNT_Level2/Vehicle/HEV_Control ==
  note: HEV Control
  Driver_demand : Inport
  HEV_sensor : Inport  Port=2
  HEV_Control : ModelReference  ModelNameDialog=HEV_Ctrl_V1_1.slx  SimulationMode=Normal  ModelReferenceVersion=1.0.47
  Rate Transition2 : RateTransition  Deterministic=off
      settings: AttributesFormatString=<Deterministic=%<Deterministic>>
  Rate Transition3 : RateTransition  Deterministic=off
      settings: AttributesFormatString=<Deterministic=%<Deterministic>>
  Rate Transition4 : RateTransition  Deterministic=off
      settings: AttributesFormatString=<Deterministic=%<Deterministic>>
  tag scope: HEV_Ctrl_PwtrCAN_Tx=scoped, HEV_ECU_Info=global
  wires:
  Driver_demand/1 -> Rate Transition3/1
  [HEV_Ctrl_PwtrCAN_Rx] -> HEV_Control/3
  HEV_sensor/1 -> Rate Transition2/1
  Rate Transition2/1 -> HEV_Control/2
  HEV_Control/2 -> Rate Transition4/1
  Rate Transition4/1 -> [HEV_ECU_Info]  "HEV_Ctrl_Info"
  HEV_Control/1 -> [HEV_Ctrl_PwtrCAN_Tx]  "HEV_Ctrl_PwtrCAN_Tx"
  Rate Transition3/1 -> HEV_Control/1

== system CtrlStrct_VNT_Level2/Vehicle/Vehicle_Motion_Control ==
  note: Vehicle Motion Control
  Env : Inport
  Rate Transition1 : RateTransition  Deterministic=off
      settings: AttributesFormatString=<Deterministic=%<Deterministic>>
  Vehicle_Motion_Control : ModelReference  ModelNameDialog=VM_Ctrl_V1_1.slx  SimulationMode=Normal  ModelReferenceVersion=0.1.24
  tag scope: VM_Ctrl_VehCAN_Tx=scoped
  wires:
  Vehicle_Motion_Control/1 -> [VM_Ctrl_VehCAN_Tx]  "VM_Ctrl_VehCAN_Tx"
  Rate Transition1/1 -> Vehicle_Motion_Control/1
  Env/1 -> Rate Transition1/1
  [VM_Ctrl_VehCAN_Rx] -> Vehicle_Motion_Control/2

== system CtrlStrct_VNT_Level2/Powertrain/Engine_Control/Engine_Control ==
  "DrvDem " : Inport
  "Eng_Sns " : Inport  Port=2
  EngineCtrl_PwtrCAN_Rx : Inport  Port=3
  "Info_in " : Inport  Port=4
  EngineCtrl_V1.slx : ModelReference  ModelNameDialog=EngineCtrl_V1_1.slx  SimulationMode=Normal  VariantControl=VarObj_EngEcu_Simple  ModelReferenceVersion=1.0.22
  EngineCtrl_V2.slx : ModelReference  ModelNameDialog=EngineCtrl_V2.slx  SimulationMode=Normal  VariantControl=VarObj_EngEcu_Medium  ModelReferenceVersion=1.0.8
  " EngineCtrl" : Outport
  " EngineCtrl_PwtrCAN_Tx" : Outport  Port=2
  " EngineCtrl_Info" : Outport  Port=3

== system CtrlStrct_VNT_Level2/Powertrain/Engine_Control/Info_in ==
  Bus Creator1 : BusCreator  Inputs=1
  Constant : Constant
  Info_in : Outport
  wires:
  Constant/1 -> Bus Creator1/1  "dummy"
  Bus Creator1/1 -> Info_in/1  "Info_in"
